simulink model "lab_1"  (R2023a)
settings: Solver=VariableStepAuto  StartTime=0.0  StopTime=10000  RelTol=1e-3  EnableMultiTasking=on
undefined symbols (not defined in the file or in its folder): QAM, qammod
libraries: commfilt2 x1, commrandsrc3 x1
settings Model: Creator=Alexey  LastModifiedBy=Дима
settings SolverCC: AlgebraicLoopSolver=TrustRegion
settings DataIOCC: ReturnWorkspaceOutputs=off
settings OptimizationCC: LifeSpan=inf
settings DebuggingCC: UnconnectedInputMsg=warning  UnconnectedOutputMsg=warning  UnconnectedLineMsg=warning  SFUnexpectedBacktrackingDiag=warning  SFNoUnconditionalDefaultTransitionDiag=warning  ArithmeticOperatorsInVariantConditions=warning
settings ModelReferenceCC: EnableRefExpFcnMdlSchedulingChecks=on
settings SFSimCC: SimUseLocalCustomCode=off  CustomCodeUndefinedFunction=UseInterfaceOnly
settings RTWCC: RTWUseLocalCustomCode=off
settings CodeAppCC: StateflowObjectComments=on
settings GRTTargetCC: TargetLangStandard=C89/C90 (ANSI)
settings ConfigComp: CovMetricSettings=dw  CovSaveCumulativeToWorkspaceVar=on  CovSaveSingleToWorkspaceVar=on  CovExternalEMLEnable=off

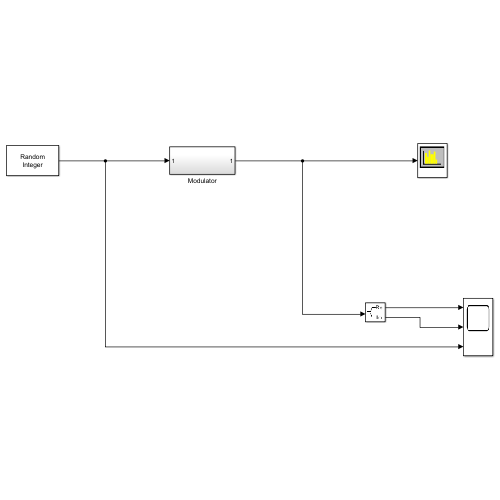
[thumbnail: Simulink's stored preview of the top-level diagram]
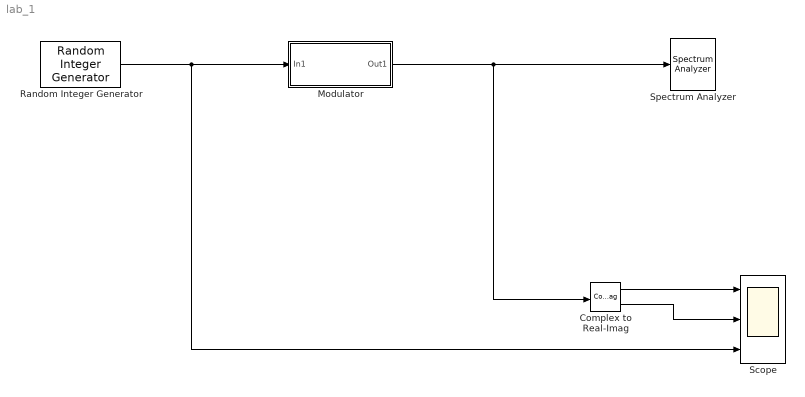
== system lab_1 ==
  Complex to Real-Imag : ComplexToRealImag
  Modulator : Subsystem
  Random Integer Generator : commrandsrc3/Random Integer Generator  SetSize=16  SeedSource=Parameter  Seed=37  SampleTime=1/9600  SamplesPerFrame=1  OutputDataType=double  SimulateUsing=Interpreted execution
  Scope : Scope  NumInputPorts=3
  Spectrum Analyzer : SpectrumAnalyzer  WindowPosition=[331 155 800 450]  Method=Welch  SampleRate=76800  AxesScaling=Manual  StartFrequency=-38400  StopFrequency=38400  FrequencyResolutionMethod=Window length  AveragingMethod=Running  YLabel=dBm  YLimits=[-108.58453410561074,20]  ShowGrid=off  DefaultConfigurationName=spbscopes.SpectrumAnalyzerBlockCfg
      settings: OpenAtSimulationStart=off
  wires:
  Random Integer Generator/1 -> Scope/3, Modulator/1(In1)
  Modulator/1(Out1) -> Complex to Real-Imag/1, Spectrum Analyzer/1
  Complex to Real-Imag/1 -> Scope/1
  Complex to Real-Imag/2 -> Scope/2

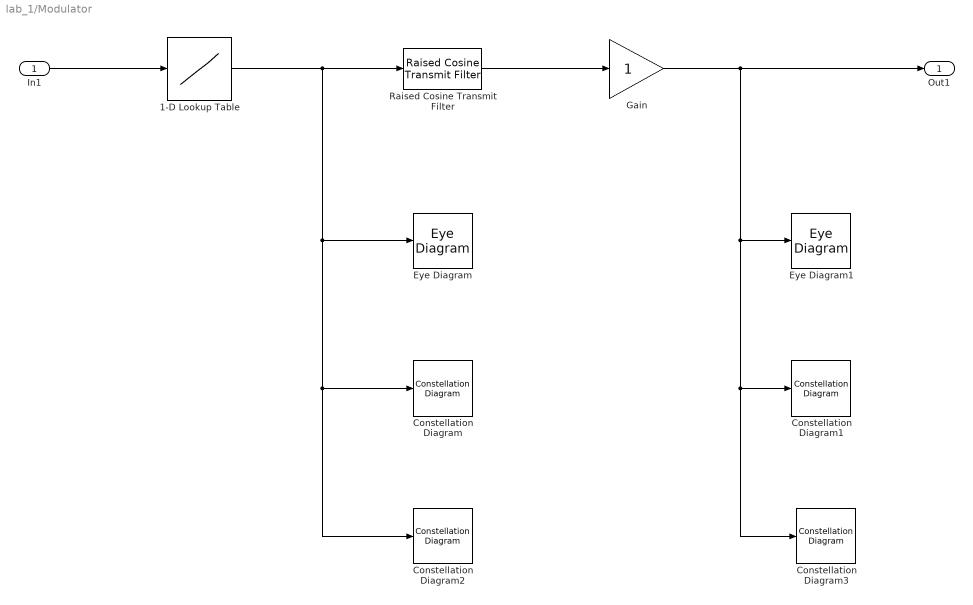
== system lab_1/Modulator ==
  In1 : Inport
  1-D Lookup Table : Lookup_n-D  NumberOfTableDimensions=1  BreakpointsForDimension1=[0:1:15]  Table=qammod([0:1:15],16)  InternalRulePriority=Speed  InputSameDT=off
  Constellation Diagram : ConstellationDiagram  WindowPosition=[512.000000,294.000000,341.000000,345.000000,]  ScopeFrameLocation=window  SymbolsToDisplaySource=Property  SymbolsToDisplay=1000  ReferenceConstellation=16-QAM  XLimits=[-3.75 3.75]  YLimits=[-3.75 3.75]  ShowTrajectory=on  DefaultConfigurationName=comm.scopes.ConstellationDiagramBlockCfg
      settings: OpenAtSimulationStart=off
  Constellation Diagram1 : ConstellationDiagram  WindowPosition=[400.000000,558.000000,601.000000,345.000000,]  ScopeFrameLocation=window  SymbolsToDisplaySource=Property  SymbolsToDisplay=1000  ReferenceConstellation=16-QAM  XLimits=[-1.9404 1.9409]  YLimits=[-1.9404 1.9409]  ShowTrajectory=on  EnableMeasurements=on  DefaultConfigurationName=comm.scopes.ConstellationDiagramBlockCfg
  Constellation Diagram2 : ConstellationDiagram  WindowPosition=[420.000000,364.000000,601.000000,345.000000,]  ScopeFrameLocation=window  SymbolsToDisplaySource=Property  SymbolsToDisplay=1000  ReferenceConstellation=16-QAM  XLimits=[-3 3]  YLimits=[-3.75 3.75]  EnableMeasurements=on  DefaultConfigurationName=comm.scopes.ConstellationDiagramBlockCfg
      settings: OpenAtSimulationStart=off
  Constellation Diagram3 : ConstellationDiagram  WindowPosition=[1016.000000,485.000000,601.000000,345.000000,]  ScopeFrameLocation=window  SymbolsToDisplaySource=Property  SymbolsToDisplay=1000  ReferenceConstellation=16-QAM  XLimits=[-1.9199 1.917]  YLimits=[-1.9199 1.917]  EnableMeasurements=on  DefaultConfigurationName=comm.scopes.ConstellationDiagramBlockCfg
      settings: OpenAtSimulationStart=off
  Eye Diagram : EyeDiagram
  Eye Diagram1 : EyeDiagram
  Gain : Gain
  Raised Cosine Transmit Filter : commfilt2/Raised Cosine Transmit Filter  filtType=Square root  R=0.8  filtSpan=10  N=8  filterGain=1  RateOptions=Allow multirate processing  framing=Mute  checkCoeff=off  variableName=rcTxFilt  checkGain=Normalized  sampMode=Mute  saveAsFlag=0  currentFiltSpan=10  D=(10)/2  launchFVT=on  roundingMode=Floor  overflowMode=off  coeffDataTypeStr=Inherit: Same word length as input  coeffMin=[]  coeffMax=[]  coeffLastDataTypeStr=Inherit: Same word length as input  outputDataTypeStr=Inherit: Same as accumulator  outputMin=[]  outputMax=[]  outputLastDataTypeStr=Inherit: Same as accumulator
  Out1 : Outport
  wires:
  Raised Cosine Transmit Filter/1 -> Gain/1
  1-D Lookup Table/1 -> Constellation Diagram2/1, Constellation Diagram/1, Eye Diagram/1, Raised Cosine Transmit Filter/1
  In1/1 -> 1-D Lookup Table/1
  Gain/1 -> Constellation Diagram3/1, Constellation Diagram1/1, Eye Diagram1/1, Out1/1
